simulink model "carrinho_duplo"  (R2013a)
settings: Solver=ode45  StartTime=0.0  StopTime=10.0  MaxStep=.1  RelTol=1e-3
values from neighbouring files (symbols this model uses):
  b1 = 1    [carrinho_duplo.m]
  b2 = 1    [carrinho_duplo.m]
  F = 4    [carrinho_duplo.m]
  k1 = 1    [carrinho_duplo.m]
  k2 = 1    [carrinho_duplo.m]
  k3 = 1    [carrinho_duplo.m]
  m1 = 1    [carrinho_duplo.m]
  m2 = 1    [carrinho_duplo.m]
  x_initial_1 = .5    (= 0.5)    [carrinho_duplo.m]
  x_initial_2 = 1    [carrinho_duplo.m]
settings Model: Creator=paulo.costa  LastModifiedBy=paulo.costa

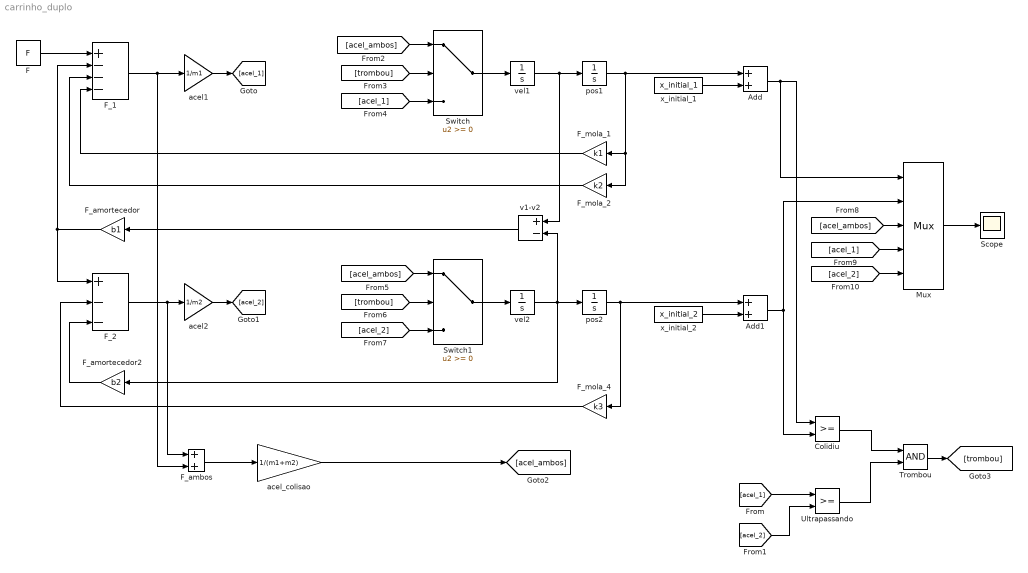
== system carrinho_duplo ==
  Add : Sum
  Add1 : Sum
  Colidiu : RelationalOperator  OutDataTypeStr=boolean
  F : Constant  Value=F
  F_1 : Sum  Inputs=+---
  F_2 : Sum  Inputs=+--
  F_ambos : Sum
  F_amortecedor : Gain  Gain=b1
  F_amortecedor2 : Gain  Gain=b2
  F_mola_1 : Gain  Gain=k1
  F_mola_2 : Gain  Gain=k2
  F_mola_4 : Gain  Gain=k3
  Mux : Mux  Inputs=5
      settings: DisplayOption=signals
  Scope : Scope
  Switch : Switch
  Switch1 : Switch
  Trombou : Logic  AllPortsSameDT=off  OutDataTypeStr=boolean
  Ultrapassando : RelationalOperator  OutDataTypeStr=boolean
  acel1 : Gain  Gain=1/m1
  acel2 : Gain  Gain=1/m2
  acel_colisao : Gain  Gain=1/(m1+m2)
  pos1 : Integrator
  pos2 : Integrator
  v1-v2 : Sum  Inputs=+-
  vel1 : Integrator
  vel2 : Integrator
  x_initial_1 : Constant  Value=x_initial_1
  x_initial_2 : Constant  Value=x_initial_2
  wires:
  F/1 -> F_1/1
  F_1/1 -> F_ambos/2, acel1/1
  vel1/1 -> v1-v2/1, pos1/1
  F_mola_1/1 -> F_1/4
  F_mola_2/1 -> F_1/3
  pos1/1 -> Add/1, F_mola_1/1, F_mola_2/1
  F_2/1 -> F_ambos/1, acel2/1
  acel2/1 -> [acel_2]
  vel2/1 -> F_amortecedor2/1, v1-v2/2, pos2/1
  pos2/1 -> Add1/1, F_mola_4/1
  v1-v2/1 -> F_amortecedor/1
  F_amortecedor/1 -> F_2/1, F_1/2
  F_mola_4/1 -> F_2/2
  F_amortecedor2/1 -> F_2/3
  x_initial_1/1 -> Add/2
  x_initial_2/1 -> Add1/2
  Add/1 -> Colidiu/1, Mux/1
  Add1/1 -> Colidiu/2, Mux/2
  Mux/1 -> Scope/1
  F_ambos/1 -> acel_colisao/1
  [acel_1] -> Ultrapassando/1
  [acel_2] -> Ultrapassando/2
  Colidiu/1 -> Trombou/1
  Ultrapassando/1 -> Trombou/2
  acel_colisao/1 -> [acel_ambos]
  Switch/1 -> vel1/1
  acel1/1 -> [acel_1]
  [trombou] -> Switch/2
  [trombou] -> Switch1/2
  Switch1/1 -> vel2/1
  Trombou/1 -> [trombou]
  [acel_1] -> Switch/3
  [acel_ambos] -> Switch/1
  [acel_2] -> Switch1/3
  [acel_ambos] -> Switch1/1
  [acel_2] -> Mux/5
  [acel_1] -> Mux/4
  [acel_ambos] -> Mux/3
